simulink subsystem "PieroControladoenPosicionz"  (R2024b)
settings: Solver=VariableStepAuto  StartTime=0.0  StopTime=10.0  RelTol=1e-3
undefined symbols (not defined in the file or in its folder): DiscIntNeverNeededParam
settings Model: Creator=claud  LastModifiedBy=claud

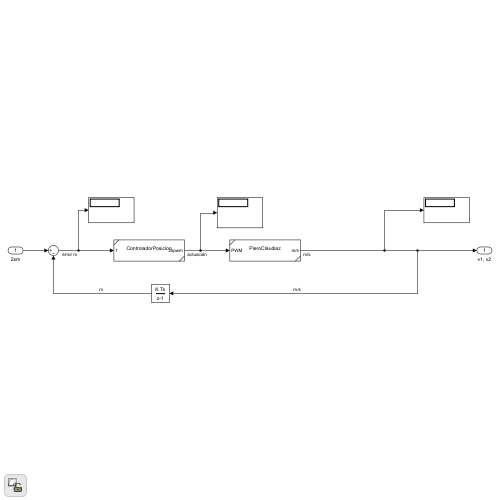
[thumbnail: Simulink's stored preview of the top-level diagram]
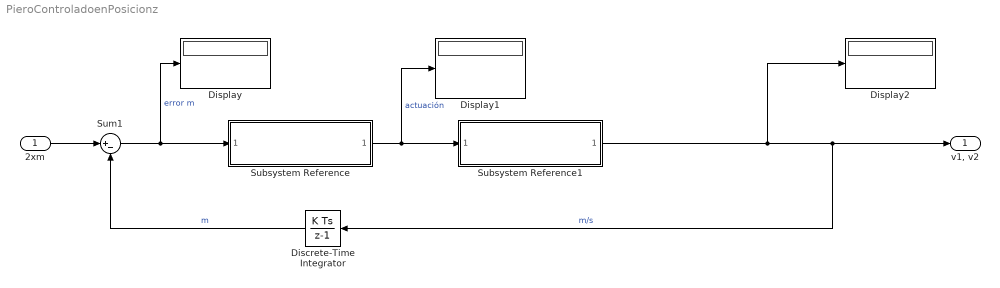
== system PieroControladoenPosicionz ==
  2xm : Inport
  Discrete-Time Integrator : DiscreteIntegrator  SampleTime=-1  ICPrevOutput=DiscIntNeverNeededParam  ICPrevScaledInput=DiscIntNeverNeededParam
  Display : Display
  Display1 : Display
  Display2 : Display
  Subsystem Reference : Subsystem  ReferencedSubsystem=ControladorPosicion
  Subsystem Reference1 : Subsystem  ReferencedSubsystem=PieroClaudiaz
  Sum1 : Sum  Inputs=|+-
  "v1, v2" : Outport
  wires:
  Discrete-Time Integrator/1 -> Sum1/2  "m"
  Subsystem Reference1/1 -> Discrete-Time Integrator/1, "v1, v2"/1, Display2/1  "m/s"
  Subsystem Reference/1 -> Display1/1, Subsystem Reference1/1  "actuación"
  2xm/1 -> Sum1/1
  Sum1/1 -> Display/1, Subsystem Reference/1  "error m"
